simulink library "cdsBitwise"  (Simulink 6.5)
libraries: simulink x1
settings Model: Creator=controls  LastModifiedBy=controls  ExtModeAutoUpdateStatusClock=off

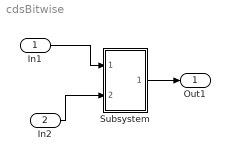
== system cdsBitwise ==
  In1 : Inport
  In2 : Inport  Port=2
  Subsystem : Subsystem
  Out1 : Outport
  wires:
  Subsystem/1(Out1) -> Out1/1
  In1/1 -> Subsystem/1(In1)
  In2/1 -> Subsystem/2(In2)

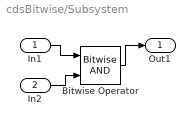
== system cdsBitwise/Subsystem ==
  In1 : Inport
  In2 : Inport  Port=2
  Bitwise Operator : simulink/Logic and Bit Operations/Bitwise Operator  logicop=AND  UseBitMask=off  NumInputPorts=2  BitMask=bin2dec('11011001')  BitMaskRealWorld=Stored Integer
  Out1 : Outport
  wires:
  In2/1 -> Bitwise Operator/2
  In1/1 -> Bitwise Operator/1
  Bitwise Operator/1 -> Out1/1
